simulink model "StateMachine_v2"  (R2015a)
settings: Solver=ode1  StartTime=0.0  StopTime=Inf  FixedStep=0.001  RelTol=1e-3
PostLoadFcn:
  | , if any(exist('dsrtsu_mdlpostloadfcn', 'file') == [2, 3, 6]), try dsrtsu_mdlpostloadfcn('Execute', bdroot); catch fprintf('Error in PostLoadFcn (dsrtsu_mdlpostloadfcn) for model "%s":\n %s\n', bdroot, lasterr); end, end,
libraries: rtican x20, rti1401lib_adc_type4 x9, rti1401lib_dio_type3 x7, rtilib1401 x1
(part 3 of 3)

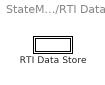
== system StateMachine_v2/RTI Data ==
  RTI Data Store : Subsystem  Tag="struct('private',struct('version',struct('dsVer',uint32(2),'dsVerCreation',uint32(2),'RTI',struct('ver','7.5','type','RTI1401')),'access',struct('type','Model','isPerm',1,'created',['26-Apr-2016 20:18:34'],'modified',['10-May-2016 14:11:22'],'location','')),'public',struct('main',struct('data',[]),'sub',struct('name',{{'StateMachine_v2'}},'data',{{struct('TH',struct('thTaskInfo',struct('taskType',{'TIMER','HWINT','TMRINT','SWINT','GLINT'},'tasksNumOf',{3,0,0,0,0},'srcIds',{{'TIMERA','TIMERA2','TIMERA3'},{},{},{},{}},'taskNames',{{['Timer Task 1'],['Timer Task 2'],['Timer Task 3']},{},{},{},{}})),'th_tc',struct('dataType',{'TASK','TASK','TASK'},'taskGroupId',{'','',''},'taskGroupList',{{},{},{}},'taskSchedulingPolicy',{'FCFS','FCFS','FCFS'},'taskType',{'TIMER','TIMER','TIMER'},'blkh',{-1,-1,-1},'srcId',{'TIMERA','TIMERA2','TIMERA3'},'srcSgnName',{['Timer A interrupt'],['Timer Task 1'],['Timer Task 1']},'srcCpuName',{'','',''},'taskName',{['Timer Task 1  [0.001] s'],['Timer Task 2  [0.01] s'],['Timer Task 3  [0.1] s']},'taskNameDisplayExt',{'','',''},'smplTime',{0.001,0.01,0.1},'smplTimeOffs',{0,0,0},'hasFixedPriority',{0,0,0},'priority',{1,2,3},'hasFixedOvc',{0,0,0},'ovcType',{1,1,1},'ovcMax',{1,1,1}),'tc_th',struct('dataType',{'TASK','TASK','TASK'},'taskGroupId',{'','',''},'taskGroupList',{{},{},{}},'taskSchedulingPolicy',{'FCFS','FCFS','FCFS'},'taskType',{'TIMER','TIMER','TIMER'},'blkh',{-1,-1,-1},'srcId',{'TIMERA','TIMERA2','TIMERA3'},'srcSgnName',{['Timer A interrupt'],['Timer Task 1'],['Timer Task 1']},'srcCpuName',{'','',''},'taskName',{['Timer Task 1  [0.001] s'],['Timer Task 2  [0.01] s'],['Timer Task 3  [0.1] s']},'taskNameDisplayExt',{'','',''},'smplTime',{0.001,0.01,0.1},'smplTimeOffs',{0,0,0},'hasFixedPriority',{0,0,0},'priority',{1,2,3},'hasFixedOvc',{0,0,0},'ovcType',{1,1,1},'ovcMax',{1,1,1}))}})))"  mask(RTI_DATA_STORE){}
      mask help:
      | RTI Data Store Block. This block is used by RTI to store internal model dependent data. Deleting this block will result in data loss.
      |
      | NEVER DELETE, COPY, OR MODIFY THIS BLOCK!
      mask Help:
      | RTI Data Store Block. This block is used by RTI to store internal model dependent data. Deleting this block will result in data loss.
      | 
      | NEVER DELETE, COPY, OR MODIFY THIS BLOCK!
      mask Display: text(0.5, 0.5, ' ', 'HorizontalAlignment', 'center');

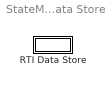
== system StateMachine_v2/RTI Data/RTI Data Store ==
  RTI Data Store : Subsystem  mask(RTI_DATA_STORE){}
      mask help:
      | RTI Data Store Block. This block is used by RTI to store internal model dependent data. Deleting this block will result in data loss.
      |
      | NEVER DELETE, COPY, OR MODIFY THIS BLOCK!
      mask Help:
      | RTI Data Store Block. This block is used by RTI to store internal model dependent data. Deleting this block will result in data loss.
      | 
      | NEVER DELETE, COPY, OR MODIFY THIS BLOCK!
      mask Display: text(0.5, 0.5, ' ', 'HorizontalAlignment', 'center');

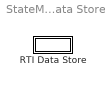
== system StateMachine_v2/RTI Data/RTI Data Store/RTI Data Store ==
  RTI Data Store : Subsystem  mask(RTI_DATA_STORE){}
      mask help:
      | RTI Data Store Block. This block is used by RTI to store internal model dependent data. Deleting this block will result in data loss.
      |
      | NEVER DELETE, COPY, OR MODIFY THIS BLOCK!
      mask Help:
      | RTI Data Store Block. This block is used by RTI to store internal model dependent data. Deleting this block will result in data loss.
      | 
      | NEVER DELETE, COPY, OR MODIFY THIS BLOCK!
      mask Display: text(0.5, 0.5, ' ', 'HorizontalAlignment', 'center');

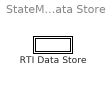
== system StateMachine_v2/RTI Data/RTI Data Store/RTI Data Store/RTI Data Store ==
  RTI Data Store : Subsystem  mask(RTI_DATA_STORE){}
      mask help:
      | RTI Data Store Block. This block is used by RTI to store internal model dependent data. Deleting this block will result in data loss.
      |
      | NEVER DELETE, COPY, OR MODIFY THIS BLOCK!
      mask Help:
      | RTI Data Store Block. This block is used by RTI to store internal model dependent data. Deleting this block will result in data loss.
      | 
      | NEVER DELETE, COPY, OR MODIFY THIS BLOCK!
      mask Display: text(0.5, 0.5, ' ', 'HorizontalAlignment', 'center');

== system StateMachine_v2/RTI Data/RTI Data Store/RTI Data Store/RTI Data Store/RTI Data Store ==

== stateflow chart StateMachine_v2/DMC1 ==
  note: dSpace en DMC krijgen stroom doordat LV switch wordt omgedraaid
  state CheckCAN
    entry: status = 0;
    entry: EnableRq = 0;
    entry: ClrErr = 0;
  note: Juiste bericht wordt opgesteld en voor de eerste keer verzonden door de dSpace
      | DMC zendt voor de eerste keer zijn berichten
  note: dSpace kijkt of hoe alle CAN berichten voor de eerste keer heeft ontvangen
  state InitialErrorClearing
    entry: status = 1;
    entry: EnableRq = 0;
    entry: ClrErr = 1;
  note: Alle berichten eens ontvangen, dus error clearen door van 0 -> 1 te zetten
  state Error
    entry: status = 2;
    entry: EnableRq = 0;
    entry: ClrErr = 0;
  note: Conditie dat beide AIRs zijn gesloten
  state ErrorFreeFrame
    state Offline
      entry: status = 4;
      entry: EnableRq = 0;
    state TimerOn
    state TimerOff
    state InitialisationRTD
      entry: status = 5;
      entry: EnableRq = 1;
      entry: ClrErr = 0;
    state RTD
      entry: status = 6;
      entry: EnableRq = 1;
    TimerOff -> Offline [order 2] : after(1,sec)
    Offline -> TimerOn : [ReadyBit == 1 && GreenButton == 1 && Brake > 50]
    TimerOn -> Offline [order 2] : [GreenButton == 0 || Brake < 50]
    TimerOn -> InitialisationRTD [order 1] : after (2,sec)
    RTD -> TimerOff : [RedButton == 1]
    TimerOff -> RTD [order 1] : [RedButton == 0]
    InitialisationRTD -> RTD : [RunningBit == 1]
  state Reset
    entry: status = 3;
    entry: EnableRq = 0;
    entry: ClrErr = 1;
  (default) -> CheckCAN
  CheckCAN -> InitialErrorClearing : [InitialMsg == 1]
  InitialErrorClearing -> Error : [after(1,sec)]
  ErrorFreeFrame -> Error : [GenErr == 1]
  Error -> Reset [order 2] : [AllowReset == 1]
  Error -> Offline [order 1] : [GenErr == 0]
  Reset -> InitialisationRTD : after(1,sec)
  data: ClrErr output; ReadyBit input; RunningBit input; GenErr input; AllowReset input; GreenButton input; RedButton input; Brake input; EnableRq output; status output; InitialMsg input

== matlab function StateMachine_v2/MATLAB Function ==
  data: u input; y output; Vin input
function y = omzetter(u,Vin)
%#codegen

y = 3435/(log((u*0.1)/(Vin-u))+11.521046)-273.15;

== stateflow chart StateMachine_v2/DMC2 ==
  note: dSpace en DMC krijgen stroom doordat LV switch wordt omgedraaid
  state CheckCAN
    entry: status = 0;
    entry: EnableRq = 0;
    entry: ClrErr = 0;
  note: Juiste bericht wordt opgesteld en voor de eerste keer verzonden door de dSpace
      | DMC zendt voor de eerste keer zijn berichten
  note: dSpace kijkt of hoe alle CAN berichten voor de eerste keer heeft ontvangen
  state InitialErrorClearing
    entry: status = 1;
    entry: EnableRq = 0;
    entry: ClrErr = 1;
  note: Alle berichten eens ontvangen, dus error clearen door van 0 -> 1 te zetten
  state Error
    entry: status = 2;
    entry: EnableRq = 0;
    entry: ClrErr = 0;
  note: Conditie dat beide AIRs zijn gesloten
  state ErrorFreeFrame
    state Offline
      entry: status = 4;
      entry: EnableRq = 0;
    state TimerOn
    state TimerOff
    state InitialisationRTD
      entry: status = 5;
      entry: EnableRq = 1;
      entry: ClrErr = 0;
    state RTD
      entry: status = 6;
      entry: EnableRq = 1;
    TimerOff -> Offline [order 2] : after(1,sec)
    Offline -> TimerOn : [ReadyBit == 1 && GreenButton == 1 && Brake > 50]
    TimerOn -> Offline [order 2] : [GreenButton == 0 || Brake < 50]
    TimerOn -> InitialisationRTD [order 1] : after (2,sec)
    RTD -> TimerOff : [RedButton == 1]
    TimerOff -> RTD [order 1] : [RedButton == 0]
    InitialisationRTD -> RTD : [RunningBit == 1]
  state Reset
    entry: status = 3;
    entry: EnableRq = 0;
    entry: ClrErr = 1;
  (default) -> CheckCAN
  CheckCAN -> InitialErrorClearing : [InitialMsg == 1]
  InitialErrorClearing -> Error : [after(1,sec)]
  ErrorFreeFrame -> Error : [GenErr == 1]
  Error -> Reset [order 2] : [AllowReset == 1]
  Error -> Offline [order 1] : [GenErr == 0]
  Reset -> InitialisationRTD : after(1,sec)
  data: ClrErr output; ReadyBit input; RunningBit input; GenErr input; AllowReset input; GreenButton input; RedButton input; Brake input; EnableRq output; status output; InitialMsg input

== matlab function StateMachine_v2/MATLAB Function1 ==
  data: u input; y output; Vin input
function y = omzetter(u,Vin)
%#codegen

y = 3435/(log((u*0.1)/(Vin-u))+11.521046)-273.15;

== matlab function StateMachine_v2/MATLAB Function2 ==
  data: u input; y output; Vin input
function y = omzetter(u,Vin)
%#codegen

y = 3435/(log((u*0.1)/(Vin-u))+11.521046)-273.15;

== matlab function StateMachine_v2/MATLAB Function3 ==
  data: u input; y output; Vin input
function y = omzetter(u,Vin)
%#codegen

y = 3435/(log((u*0.1)/(Vin-u))+11.521046)-273.15;

== matlab function StateMachine_v2/MATLAB Function4 ==
  data: u input; y output; Vin input
function y = omzetter(u,Vin)
%#codegen

y = 3435/(log((u*0.1)/(Vin-u))+11.521046)-273.15;

== matlab function StateMachine_v2/MATLAB Function5 ==
  data: u input; y output; Vin input
function y = omzetter(u,Vin)
%#codegen

y = 3435/(log((u*0.1)/(Vin-u))+11.521046)-273.15;

== matlab function StateMachine_v2/MATLAB Function6 ==
  data: u input; y output; Vin input
function y = omzetter(u,Vin)
%#codegen

y = 3435/(log((u*0.1)/(Vin-u))+11.521046)-273.15;

== matlab function StateMachine_v2/MATLAB Function7 ==
  data: u input; y output; Vin input
function y = omzetter(u,Vin)
%#codegen

y = 3435/(log((u*0.1)/(Vin-u))+11.521046)-273.15;
